simulink model "c166_bitfields"  (Simulink 6.0)
settings: Solver=FixedStepDiscrete  StartTime=0.0  StopTime=10.0  FixedStep=1.0  RelTol=1e-3
PostLoadFcn:
  | c166bitfielddata
values from neighbouring files (symbols this model uses):
  rpmCheckEnabled = SimulinkC166.Parameter    [c166bitfielddata.m]
  rpmLimit = uint16(500)    [c166bitfielddata.m]
  tempCheckEnabled = SimulinkC166.Parameter    [c166bitfielddata.m]
  tempLimit = uint16(500)    [c166bitfielddata.m]
settings Model: CovMetricSettings=d  Creator=The MathWorks Inc.  LastModifiedBy=batserve  ExtModeAutoUpdateStatusClock=off  ProdHWDeviceType=Infineon C16x
settings DataIOCC: SaveFormat=Structure  SignalLoggingName=sigsOut
settings OptimizationCC: InlineParams=on  ZeroExternalMemoryAtStartup=off  ZeroInternalMemoryAtStartup=off  InitFltsAndDblsToZero=off  LifeSpan=1
settings DebuggingCC: CheckExecutionContextPreStartOutputMsg=on  CheckExecutionContextRuntimeOutputMsg=on  SolverPrmCheckMsg=none
settings HardwareCC: ProdBitPerInt=16  ProdEndianess=LittleEndian  ProdWordSize=16  ProdHWDeviceType=Infineon C16x  TargetHWDeviceType=32-bit Generic
settings RTWCC: SystemTargetFile=c166.tlc  TemplateMakefile=c166.tmf  GenerateReport=on  ProcessScript=c166_make_rtw_hook  LaunchReport=on
settings CodeAppCC: IgnoreCustomStorageClasses=off  PrefixModelToSubsysFcnNames=off
settings STFCustomTargetCC: TargetFcnLib=ansi_tfl_tmw.mat  GenFloatMathFcnCalls=ANSI_C  GenerateSampleERTMain=on  IncludeMdlTerminateFcn=off  CombineOutputUpdateFcns=on  ERTCustomFileBanners=on  SupportNonFinite=off  SupportComplex=off  PurelyIntegerCode=on  SystemTargetFile=c166.tlc
settings ERTTargetCC: TargetFcnLib=ansi_tfl_tmw.mat  GenFloatMathFcnCalls=ANSI_C  GenerateSampleERTMain=on  IncludeMdlTerminateFcn=off  SupportNonFinite=off  SupportComplex=off  PurelyIntegerCode=on  SupportContinuousTime=on  SupportNonInlinedSFcns=on  RootIOFormat=Individual Arguments  ERTCustomFileTemplate=example_file_process.tlc  InitialValueSource=Model
settings CustomProperty: DataType=RTWOptions_EnumType__toolbox_rtw_targets_c166_c166_c166_BuildActionC166  Value=Run_with_simulator
settings EnumStrPairs: String=Run_with_simulator

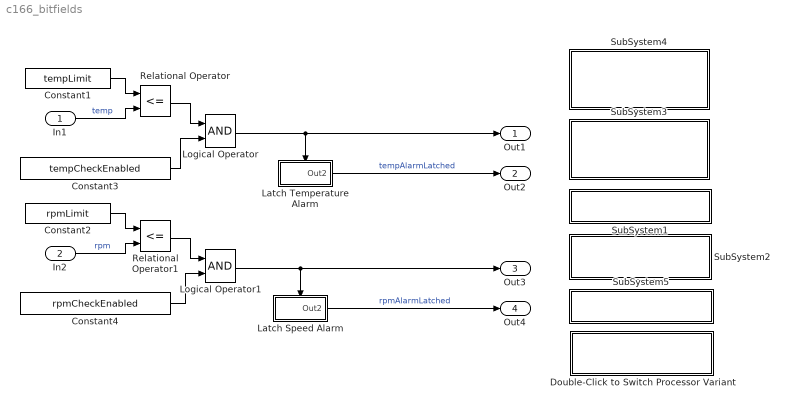
== system c166_bitfields ==
  In1 : Inport  Port=1  DataType=uint16  LatchInput=off
  In2 : Inport  Port=2  DataType=uint16  LatchInput=off
  Constant1 : Constant  Value=tempLimit
  Constant2 : Constant  Value=rpmLimit
  Constant3 : Constant  Value=tempCheckEnabled
  Constant4 : Constant  Value=rpmCheckEnabled
  Double-Click to Switch Processor Variant : Subsystem  PropExecContextAcrossSSBoundary=on
      settings: OpenFcn=c166switchconfig(gcs)
      mask Display: disp('Switch Target\nProcessor Variant');
  Latch Speed Alarm : Subsystem  PropExecContextAcrossSSBoundary=on
  Latch Temperature Alarm : Subsystem  PropExecContextAcrossSSBoundary=on
  Logical Operator : Logic  AllPortsSameDT=off
  Logical Operator1 : Logic  AllPortsSameDT=off
  Relational Operator : RelationalOperator  Operator=<=
  Relational Operator1 : RelationalOperator  Operator=<=
  SubSystem1 : Subsystem  PropExecContextAcrossSSBoundary=on
      settings: OpenFcn=rtwprivate daexplrwsview;
      mask Display: disp('Inspect data objects');
  SubSystem2 : Subsystem  PropExecContextAcrossSSBoundary=on
      settings: OpenFcn=|
      | uset_param(gcs,'BuildActionC166','Run_with_simulator');
      | make_rtw
      mask Display: disp('Generate code and\nlaunch debugger');
  SubSystem3 : Subsystem  PropExecContextAcrossSSBoundary=on
      settings: OpenFcn=helpview([docroot,'/toolbox/ecoder/ecoder.map'], 'rtw_custom_storage')
      mask Display: disp('Read documentation\n for custom\nstorage classes');
  SubSystem4 : Subsystem  PropExecContextAcrossSSBoundary=on
      settings: OpenFcn=helpview([docroot,'/toolbox/c166/c166.map'], 'c166_bit_addressable')
      mask Display: disp('Read documentation\nfor C166 bit-\naddressable memory')
  SubSystem5 : Subsystem  PropExecContextAcrossSSBoundary=on
      settings: OpenFcn=edit c166bitfielddata.m
      mask Display: disp('Open setup file');
  Out1 : Outport
  Out2 : Outport  Port=2
  Out3 : Outport  Port=3
  Out4 : Outport  Port=4
  wires:
  In1/1 -> Relational Operator/2  "temp"
  Constant1/1 -> Relational Operator/1
  Relational Operator/1 -> Logical Operator/1
  Latch Temperature Alarm/1(Out2) -> Out2/1  "tempAlarmLatched"
  In2/1 -> Relational Operator1/2  "rpm"
  Constant2/1 -> Relational Operator1/1
  Relational Operator1/1 -> Logical Operator1/1
  Latch Speed Alarm/1(Out2) -> Out4/1  "rpmAlarmLatched"
  Logical Operator/1 -> Out1/1, Latch Temperature Alarm/Enable
  Logical Operator1/1 -> Out3/1, Latch Speed Alarm/Enable
  Constant3/1 -> Logical Operator/2
  Constant4/1 -> Logical Operator1/2

== system c166_bitfields/Double-Click to Switch Processor Variant ==

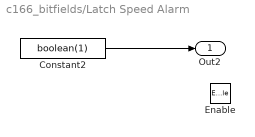
== system c166_bitfields/Latch Speed Alarm ==
  Enable : EnablePort
  Constant2 : Constant  Value=boolean(1)
  Out2 : Outport  InitialOutput=0
  wires:
  Constant2/1 -> Out2/1

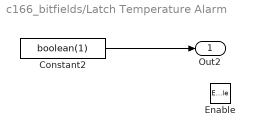
== system c166_bitfields/Latch Temperature Alarm ==
  Enable : EnablePort
  Constant2 : Constant  Value=boolean(1)
  Out2 : Outport  InitialOutput=0
  wires:
  Constant2/1 -> Out2/1

== system c166_bitfields/SubSystem1 ==

== system c166_bitfields/SubSystem2 ==

== system c166_bitfields/SubSystem3 ==

== system c166_bitfields/SubSystem4 ==

== system c166_bitfields/SubSystem5 ==
